simulink model "combFilterFeedforward"  (R2022a)
settings: Solver=FixedStepDiscrete  StartTime=0.0  StopTime=simParams.stopTime  RelTol=1e-3
PostLoadFcn:
  | postLoadCallback
InitFcn:
  | initCallback
StopFcn:
  | stopCallback
undefined symbols (not defined in the file or in its folder): modelParams
libraries: dspsrcs4 x5
CloseFcn:
  | closeCallback
settings Model: DataTypeOverride=Off  SimulationMode=accelerator  Creator=Ross_admin  LastModifiedBy=trevvvy
settings DataIOCC: ReturnWorkspaceOutputs=off
settings OptimizationCC: BlockReduction=off  ConditionallyExecuteInputs=off  DefaultParameterBehavior=Inlined
settings DebuggingCC: AlgebraicLoopMsg=error  SingleTaskRateTransMsg=error  UnconnectedInputMsg=warning  UnconnectedOutputMsg=warning  UnconnectedLineMsg=warning
settings HardwareCC: ProdBitPerPointer=32  ProdBitPerSizeT=32  ProdBitPerPtrDiffT=32  ProdLargestAtomicFloat=None  ProdIntDivRoundTo=Undefined  ProdEndianess=Unspecified  ProdWordSize=32  ProdHWDeviceType=ASIC/FPGA->ASIC/FPGA  TargetBitPerLong=64  TargetBitPerPointer=64  TargetBitPerSizeT=64  TargetBitPerPtrDiffT=64  TargetLongLongMode=on  TargetIntDivRoundTo=Zero  TargetEndianess=LittleEndian  TargetWordSize=64  TargetHWDeviceType=Custom Processor->MATLAB Host Computer  ProdEqTarget=off
settings RTWCC: DLArmComputeVersion=19.05

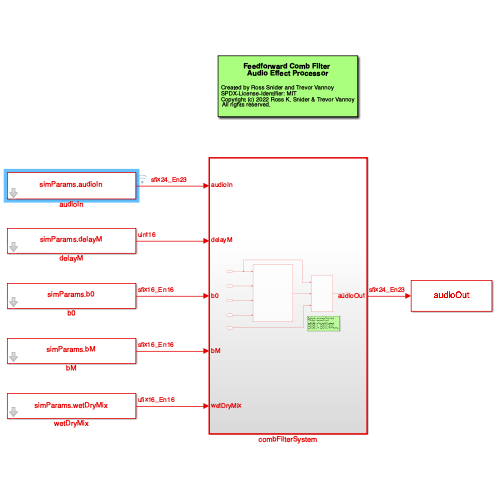
[thumbnail: Simulink's stored preview of the top-level diagram]
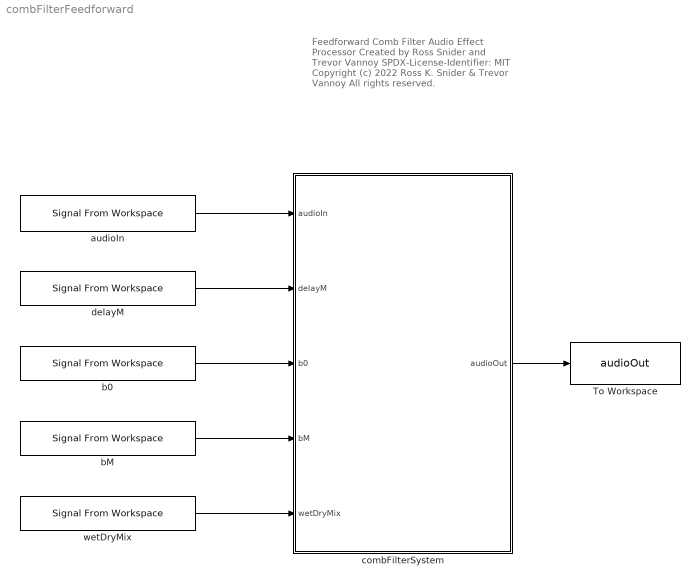
== system combFilterFeedforward ==
  note: Feedforward Comb Filter
      | Audio Effect Processor
      |
      | Created by Ross Snider and Trevor Vannoy
      | SPDX-License-Identifier: MIT
      | Copyright (c) 2022 Ross K. Snider & Trevor Vannoy
      | All rights reserved.
  To Workspace : ToWorkspace  VariableName=audioOut  SampleTime=-1
      settings: Save2DSignal=2-D array (concatenate along first dimension)
  audioIn : dspsrcs4/Signal From Workspace  X=simParams.audioIn  Ts=modelParams.audio.samplePeriod  nsamps=1  OutputAfterFinalValue=Setting to zero  ignoreOrWarnInputAndFrameLengths=off  OutputFrames=off
  b0 : dspsrcs4/Signal From Workspace  X=simParams.b0  Ts=modelParams.audio.samplePeriod  nsamps=1  OutputAfterFinalValue=Holding final value  ignoreOrWarnInputAndFrameLengths=off  OutputFrames=off
  bM : dspsrcs4/Signal From Workspace  X=simParams.bM  Ts=modelParams.audio.samplePeriod  nsamps=1  OutputAfterFinalValue=Holding final value  ignoreOrWarnInputAndFrameLengths=off  OutputFrames=off
  combFilterSystem : Subsystem  TreatAsAtomicUnit=on
  delayM : dspsrcs4/Signal From Workspace  X=simParams.delayM  Ts=modelParams.audio.samplePeriod  nsamps=1  OutputAfterFinalValue=Holding final value  ignoreOrWarnInputAndFrameLengths=off  OutputFrames=off
  wetDryMix : dspsrcs4/Signal From Workspace  X=simParams.wetDryMix  Ts=modelParams.audio.samplePeriod  nsamps=1  OutputAfterFinalValue=Holding final value  ignoreOrWarnInputAndFrameLengths=off  OutputFrames=off
  wires:
  combFilterSystem/1(audioOut) -> To Workspace/1
  audioIn/1 -> combFilterSystem/1(audioIn)
  wetDryMix/1 -> combFilterSystem/5(wetDryMix)
  delayM/1 -> combFilterSystem/2(delayM)
  b0/1 -> combFilterSystem/3(b0)
  bM/1 -> combFilterSystem/4(bM)

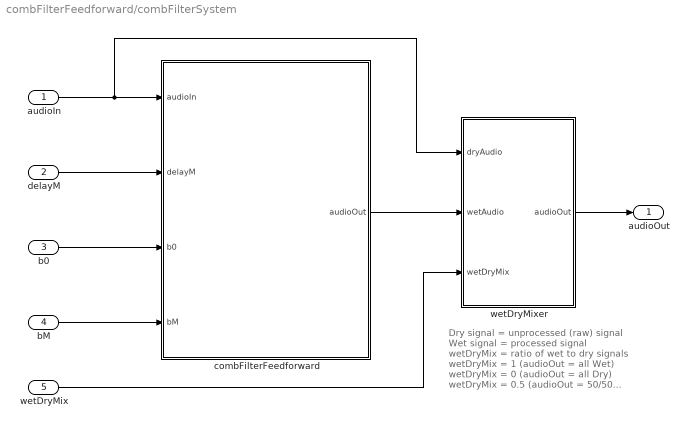
== system combFilterFeedforward/combFilterSystem ==
  note: Dry signal = unprocessed (raw) signal
      | Wet signal = processed signal
      |
      | wetDryMix = ratio of wet to dry signals
      | wetDryMix = 1 (audioOut = all Wet)
      | wetDryMix = 0 (audioOut = all Dry)
      | wetDryMix = 0.5 (audioOut = 50/50 Wet/Dry)
  audioIn : Inport
  delayM : Inport  Port=2
  b0 : Inport  Port=3
  bM : Inport  Port=4
  wetDryMix : Inport  Port=5
  combFilterFeedforward : Subsystem
  wetDryMixer : Subsystem
  audioOut : Outport
  wires:
  delayM/1 -> combFilterFeedforward/2(delayM)
  combFilterFeedforward/1(audioOut) -> wetDryMixer/2(wetAudio)
  audioIn/1 -> wetDryMixer/1(dryAudio), combFilterFeedforward/1(audioIn)
  wetDryMixer/1(audioOut) -> audioOut/1
  b0/1 -> combFilterFeedforward/3(b0)
  bM/1 -> combFilterFeedforward/4(bM)
  wetDryMix/1 -> wetDryMixer/3(wetDryMix)

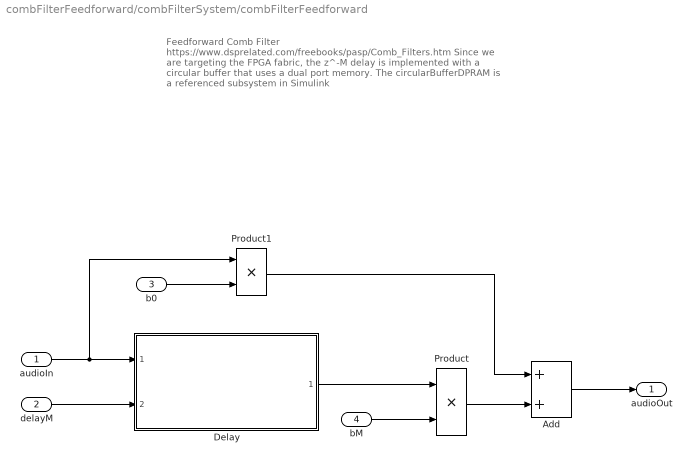
== system combFilterFeedforward/combFilterSystem/combFilterFeedforward ==
  note: Feedforward Comb Filter
      |
      | https://www.dsprelated.com/freebooks/pasp/Comb_Filters.htm
      |
      | Since we are targeting the FPGA fabric, the z^-M delay is implemented with a circular buffer that uses a
      | dual port memory. The circularBufferDPRAM is a
      | referenced subsystem in Simulink
  audioIn : Inport
  delayM : Inport  Port=2
  b0 : Inport  Port=3
  bM : Inport  Port=4
  Add : Sum  OutDataTypeStr=fixdt(1, modelParams.audio.wordLength, modelParams.audio.fractionLength)  SaturateOnIntegerOverflow=on
  Delay : Subsystem  ReferencedSubsystem=circularBufferDPRAM
  Product : Product  OutDataTypeStr=fixdt(1, modelParams.audio.wordLength, modelParams.audio.fractionLength)
  Product1 : Product  OutDataTypeStr=fixdt(1, modelParams.audio.wordLength, modelParams.audio.fractionLength)
  audioOut : Outport
  wires:
  audioIn/1 -> Product1/1, Delay/1
  Delay/1 -> Product/1
  Product1/1 -> Add/1
  Add/1 -> audioOut/1
  b0/1 -> Product1/2
  delayM/1 -> Delay/2
  bM/1 -> Product/2
  Product/1 -> Add/2

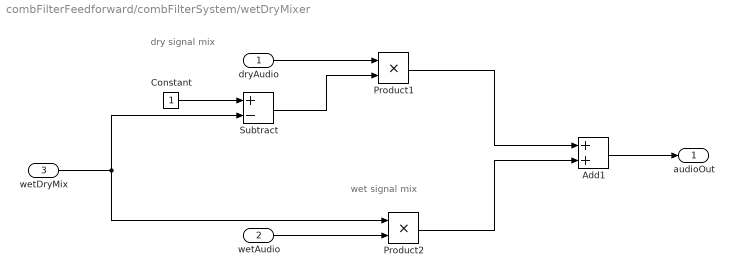
== system combFilterFeedforward/combFilterSystem/wetDryMixer ==
  note: wet signal mix
  note: dry signal mix
  dryAudio : Inport
  wetAudio : Inport  Port=2
  wetDryMix : Inport  Port=3
  Add1 : Sum  OutDataTypeStr=fixdt(1, modelParams.audio.wordLength, modelParams.audio.fractionLength)  SaturateOnIntegerOverflow=on
  Constant : Constant  OutDataTypeStr=fixdt(0,1,0)  SampleTime=modelParams.audio.samplePeriod
  Product1 : Product  OutDataTypeStr=fixdt(1, modelParams.audio.wordLength, modelParams.audio.fractionLength)
  Product2 : Product  OutDataTypeStr=fixdt(1, modelParams.audio.wordLength, modelParams.audio.fractionLength)
  Subtract : Sum  Inputs=+-  OutDataTypeStr=fixdt(1,modelParams.audio.wordLength,modelParams.audio.fractionLength)
  audioOut : Outport
  wires:
  Product2/1 -> Add1/2
  Add1/1 -> audioOut/1
  Product1/1 -> Add1/1
  Constant/1 -> Subtract/1
  wetAudio/1 -> Product2/2
  Subtract/1 -> Product1/2
  wetDryMix/1 -> Product2/1, Subtract/2
  dryAudio/1 -> Product1/1
